simulink library "test"  (Simulink 3.00)
PostLoadFcn:
  | setsysloc simulink_extras
undefined symbols (not defined in the file or in its folder): A, B, C, D, Dd, den, num, offset, sfuncorr, sfunpsd
settings Model: Creator=ldean  LastModifiedBy=jon

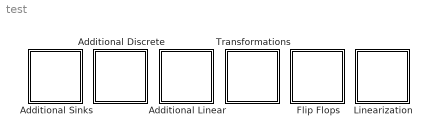
== system test ==
  Additional Discrete : Subsystem
      mask Display: plot([-20 20],[-15 -15],[-15 -15],[-20 20], [ -15  -10  -10 -5 -5  0  0 5 5 10 10 15 15 20],[-10 -10 2  2  13 13 8  8  4  4  1  1  -1 -1])
  Additional Linear : Subsystem
      mask Display: plot([-20 20],[-15 -15],[-15 -15],[-20 20],[-20 20],[-5 18])
  Additional Sinks : Subsystem
      mask Display:
      | plot([-1 1 1 -1 1],[ 1 -1 1 -1 1],[14 4 11 4 6],[14 4 6 4 11],[14 4 11 4 6],[-14 -4 -6 -4 -11],[-14 -4 -11 -4 -6],[14 4 6 4 11],[-14 -4 -11 -4 -6],[-14 -4 -6 -4 -11],
      | [0 0 3 0 -3],[-20 -5 -10 -5 -10],[0 0 3 0 -3],[20 5 10 5 10],[20 5 10 5 10],[0 0 3 0 -3],[-20 -5 -10 -5 -10],[0 0 3 0 -3])
  Flip Flops : Subsystem
  Linearization : Subsystem
  Transformations : Subsystem

== system test/Additional Discrete ==
  Discrete Transfer Fcn (with initial outputs) : Subsystem  mask(Discrete Transfer Function with Initial Outputs){N=[1], D=[1  .5], U0=[1], Y0=-.5, TS=1}
      mask prompts: N "Numerator:"; D "Denominator:"; U0 "Initial input:"; Y0 "Initial output:"; TS "Sample time:"
      mask help: Vector expressions for numerator, and denominator. Coefficients are in descending powers of z.
      mask init:
      | [A,B,C,Dd]=tf2ss(N,D);if (isempty(Y0));[m,n]=size(A);X0=zeros(1,m); end;if (isempty(U0));[m,p]=size(B);U0=zeros(1,p);end;X0=getxo(A,B,C,Dd,U0,Y0,1);
      mask Help: Specify the initial output for the transfer function.  An optimization routine attempts to determine the appropriate initial states so that the specified initial output is achieved.  For more details, see the m-file getxo.m
      mask Display: dpoly(N,D,'z')
  Discrete Transfer Fcn (with initial states) : Subsystem  mask(Discrete Transfer Function with Initial States){N=[1], D=[1  .5], X0=[1], TS=.5}
      mask prompts: N "Numerator:"; D "Denominator:"; X0 "Initial conditions:"; TS "Sample time:"
      mask help: Vector expressions for numerator, and denominator. Coefficients are in descending powers of z.
      mask init:
      | [A,B,C,Dd]=tf2ss(N,D);if (isempty(X0));[m,n]=size(A);X0=zeros(1,m); end;
      mask Help: Specify the initial states for the transfer function.  The state ordering is determined by the m-file tf2ss.  There is no unique mapping of the states in a transfer function to states in a state-space representation.  However, tf2ss will consistently use the same mapping for a given transfer function.
      mask Display: dpoly(N,D,'z')
  Discrete Zero-Pole (with initial outputs) : Subsystem  mask(Discrete Zero-Pole with Initial Outputs){Z=[1], P=[0  .5], K=[1], U0=1, Y0=.5, TS=1}
      mask prompts: Z "Zeros:"; P "Poles:"; K "Gain:"; U0 "Initial input:"; Y0 "Initial output:"; TS "Sample time:"
      mask help: Vector expressions for numerator, denominator, and gain.
      mask init:
      | [A,B,C,D]=zp2ss(Z,P,K);if (isempty(Y0));[m,n]=size(A);X0=zeros(1,m); end;if (isempty(U0));[m,p]=size(B);U0=zeros(1,p);end;X0=getxo(A,B,C,D,U0,Y0,1);
      mask Help: Specify the initial output for the zero-pole-gain system.  An optimization routine attempts to determine the appropriate initial states so that the specified initial output is achieved.  For more details, see the m-file getxo.m
      mask Display: droots(Z,P,K,'z')
  Discrete Zero-Pole (with initial states) : Subsystem  mask(Discrete Zero-Pole with Initial States){Z=[1], P=[0  .5], K=[1], X0=1, TS=.5}
      mask prompts: Z "Zeros:"; P "Poles:"; K "Gain:"; X0 "Initial conditions:"; TS "Sample time:"
      mask help: Vector expressions for numerator, denominator, and gain.
      mask init:
      | [A,B,C,D]=zp2ss(Z,P,K);if (isempty(X0));[m,n]=size(A);X0=zeros(1,m); end;
      mask Help: Specify the initial states for the transfer function.  The state ordering is determined by the m-file zp2ss.  There is no unique mapping of the states in a zero-pole-gain representation to states in a state-space representation.  However, zp2ss will consistently use the same mapping for a given transfer function.
      mask Display: droots(Z,P,K,'z')

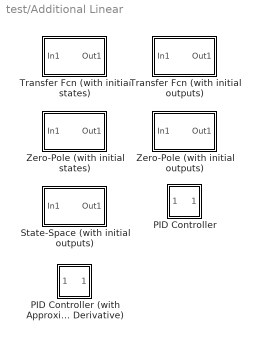
== system test/Additional Linear ==
  PID Controller : Subsystem  mask(PID Controller){P=1, I=1, D=0}
      mask prompts: P "Proportional:"; I "Integral:"; D "Derivative:"
      mask help:
      | Enter expressions for proportional, integral, and derivative terms.
      | P+I/s+Ds
      mask Help: This block implements a PID controller where parameters are entered for the Proportional, Integral and Derivative terms. Unmask this block to see how it works. The derivative term is implemented using a true derivative block.
      mask Display: disp('PID')
  PID Controller (with Approximate Derivative) : Subsystem  mask(PID(2) Controller){P=1, I=1, D=0, N=100}
      mask prompts: P "Proportional:"; I "Integral:"; D "Derivative:"; N "Derivative divisor(N):"
      mask help:
      | Enter Proportional(P), Integral(I), and Derivative(D) and divisor (N) terms.
      | P+I/s+Ds/(1/Ns+1)
      mask Help: This block implements a PID controller where parameters are entered for the Proportional, Integral and Derivative and divisor terms. Unmask this block to see how it works. The derivative term is implemented using an s/(s/N +1)  transfer function block. Making N large can create a "stiff" system.
      mask Display: disp('PID')
  State-Space (with initial outputs) : Subsystem  mask(State-Space with Initial Outputs){A=[-2.0479 -.4517;-.4517 -3.0295], B=[.0591 0]', C=[.2641 .8717], D=0, U0=1, Y0=.5}
      mask prompts: U0 "Initial inputs:"; Y0 "Initial outputs:"
      mask help:
      | State-Space model matrices:
      | dx/dt = Ax + Bu
      | y=Cx +Du
      mask init:
      | if (isempty(Y0));[m,n]=size(A);X0=zeros(1,m); end; if (isempty(U0));[m,p]=size(B);U0=zeros(1,p);end;X0=getxo(A,B,C,D,U0,Y0,0);
      mask Help: Specify an initial output.  An optimization routine is used to attempt to find the steady state x values that satisfy the initial output.  The block states will be initialized to these values.
      mask Display: fprintf('x'' = Ax + Bu\n  y = Cx + Du');
  Transfer Fcn (with initial outputs) : Subsystem  mask(Transfer Function with Initial Outputs){N=[1], D=[1  1], Y0=.5, U0=0}
      mask prompts: N "Numerator:"; D "Denominator:"; Y0 "Initial output:"; U0 "Initial input:"
      mask help: Vector expressions for numerator, and denominator. Coefficients are in descending powers of s.
      mask init:
      | [A,B,C,Dd]=tf2ss(N,D);if (isempty(Y0));[m,n]=size(A);X0=zeros(1,m); end; if (isempty(U0));[m,p]=size(B);U0=zeros(1,p);end;X0=getxo(A,B,C,Dd,U0,Y0,0);
      mask Help: Specify the initial output for the transfer function.  An optimization routine attempts to determine the appropriate initial states so that the specified initial output is achieved.  For more details, see the m-file getxo.m
      mask Display: dpoly(N,D,'s')
  Transfer Fcn (with initial states) : Subsystem  mask(Transfer Function with Initial States){N=[1], D=[1  1], X0=.5}
      mask prompts: N "Numerator:"; D "Denominator:"; X0 "Initial conditions:"
      mask help: Vector expressions for numerator, and denominator. Coefficients are in descending powers of s.
      mask init:
      | [A,B,C,Dd]=tf2ss(N,D);if (isempty(X0));[m,n]=size(A);X0=zeros(1,m); end;
      mask Help: Specify the initial states for the transfer function.  The state ordering is determined by the m-file tf2ss.  There is no unique mapping of the states in a transfer function to states in a state-space representation.  However, tf2ss will consistently use the same mapping for a given transfer function.
      mask Display: dpoly(N,D,'s')
  Zero-Pole (with initial outputs) : Subsystem  mask(Zero-Pole with Initial Outputs){Z=[1], P=[0; -1], K=[1], Y0=.5, U0=0}
      mask prompts: Z "Zeros:"; P "Poles:"; K "Gain:"; Y0 "Initial output:"; U0 "Initial input:"
      mask help: Vector expressions for numerator, denominator, and gain.
      mask init:
      | [A,B,C,D]=zp2ss(Z,P,K);if (isempty(Y0));[m,n]=size(A);X0=zeros(1,m); end; if (isempty(U0));[m,p]=size(B);U0=zeros(1,p);end;X0=getxo(A,B,C,D,U0,Y0,0);
      mask Help: Specify the initial output for the zero-pole-gain system.  An optimization routine attempts to determine the appropriate initial states so that the specified initial output is achieved.  For more details, see the m-file getxo.m
      mask Display: droots(Z,P,K)
  Zero-Pole (with initial states) : Subsystem  mask(Zero-Pole with Initial States){Z=[1], P=[0; -1], K=[1], X0=.5}
      mask prompts: Z "Zeros:"; P "Poles:"; K "Gain:"; X0 "Initial conditions:"
      mask help: Vector expressions for numerator, denominator, and gain.
      mask init:
      | [A,B,C,D]=zp2ss(Z,P,K);if (isempty(X0));[m,n]=size(A);X0=zeros(1,m); end;
      mask Help: Specify the initial states for the transfer function.  The state ordering is determined by the m-file zp2ss.  There is no unique mapping of the states in a zero-pole-gain representation to states in a state-space representation.  However, zp2ss will consistently use the same mapping for a given transfer function.
      mask Display: droots(Z,P,K)

== system test/Additional Sinks ==
  Auto Correlator : Subsystem  LoadFcn=sfuncorr([],[],[],'LoadBlock')  StartFcn=sfuncorr([],[],[],'Start')  mask(Auto Correlator){npts=100, HowOften=50, sampleT=0.1}
      mask prompts: npts "Length of buffer:"; HowOften "Plot after how many points:"; sampleT "Sample time:"
      mask help:
      | Auto correlator using graph window.
      | Requires signal processing toolbox.
      mask init:
      | ts=sampleT(1); if length(sampleT) > 1, offset = sampleT(2);, else, offset = 0; end
      settings: CopyFcn=sfuncorr([],[],[],'CopyBlock')  DeleteFcn=sfuncorr([],[],[],'DeleteBlock')  NameChangeFcn=sfuncorr([],[],[],'NameChange')
      mask Help: This block when hooked to the output of a system displays the auto correlation of the buffer in the graph window. For more see the M-file sfuncorr.
      mask Display: plot(0,0,100,100,[11,93,93,11,11],[90,90,40,40,90],[80,60,40,20],[50,79,50,80])
  Averaging Power Spectral Density : Subsystem  LoadFcn=sfunpsd([],[],[],'LoadBlock')  StartFcn=sfunpsd([],[],[],'Start')  mask(Spectrum Analyzer){npts=128, fftpts=512, HowOften=64, sampleT=0.1}
      mask prompts: npts "Length of buffer:"; fftpts "Number of points for fft:"; HowOften "Plot after how many points:"; sampleT "Sample time:"
      mask help: Spectrum analyzer using graph window.
      mask init:
      | ts=sampleT(1); if length(sampleT) > 1, offset = sampleT(2);, else, offset = 0; end
      settings: CopyFcn=sfunpsd([],[],[],'CopyBlock')  DeleteFcn=sfunpsd([],[],[],'DeleteBlock')  NameChangeFcn=sfunpsd([],[],[],'NameChange')
      mask Help: This block when hooked to the output of a system displays the frequency content of the buffer in the graph window. For more see the M-file sfunpsd.
      mask Display: plot(0,0,100,100,[11,92,92,11,11],[90,90,40,40,90],[82,76,65,57,51,44,35,30,25,20],[65,62,59,63,66,66,67,70,55,50])
  Averaging Spectrum Analyzer : Subsystem  mask(Spectrum Analyzer){npts=256, fftpts=256, HowOften=64, sampleT=0.1}
      mask prompts: npts "Length of buffer:"; fftpts "Number of points for fft:"; HowOften "Plot after how many points:"; sampleT "Sample time:"
      mask help:
      | Spectrum analyser using graph window.
      | Hook input 1 to system input.
      | Hook input 2 to system output.
      mask init:
      | ts=sampleT(1); if length(sampleT) > 1, offset = sampleT(2);, else, offset = 0; end
      mask Help: Hook the system's input to the first port of this block and the system's output to second port. Results are displayed as the frequency response of this system. Use signals with high harmonic content for best results.
      mask Display: plot(0,0,100,100,[12,92,92,12,12],[90,90,40,40,90],[80,72,63,54,47,40,32,20],[61,61,62,65,69,73,75,75])
  Cross Correlator : Subsystem  LoadFcn=sfuncorr([],[],[],'LoadBlock')  StartFcn=sfuncorr([],[],[],'Start')  mask(Cross Correlator){npts=100, HowOften=50, sampleT=0.1}
      mask prompts: npts "Length of buffer:"; HowOften "Plot after how many points:"; sampleT "Sample time:"
      mask help:
      | Cross correlator using graph window.
      | Requires signal processing toolbox.
      mask init:
      | ts=sampleT(1); if length(sampleT) > 1, offset = sampleT(2);, else, offset = 0; end
      settings: CopyFcn=sfuncorr([],[],[],'CopyBlock')  DeleteFcn=sfuncorr([],[],[],'DeleteBlock')  NameChangeFcn=sfuncorr([],[],[],'NameChange')
      mask Help: This block when hooked to the outputs of a system displays the cross correlation of the buffer in the graph window. For more see the M-file sfuncorr.
      mask Display: plot(0,0,100,100,[10,92,92,10,10],[90,90,40,40,90],[80,59,40,20],[70,79,70,79],[79,70,59,51,40,30,21],[60,51,60,50,60,50,60])
  Power Spectral Density : Subsystem  LoadFcn=sfunpsd([],[],[],'LoadBlock')  StartFcn=sfunpsd([],[],[],'Start')  mask(Spectrum Analyzer){npts=128, fftpts=512, HowOften=64, sampleT=0.1}
      mask prompts: npts "Length of buffer:"; fftpts "Number of points for fft:"; HowOften "Plot after how many points:"; sampleT "Sample time:"
      mask help: Spectrum analyser using graph window.
      mask init:
      | ts=sampleT(1); if length(sampleT) > 1, offset = sampleT(2);, else, offset = 0; end
      settings: CopyFcn=sfunpsd([],[],[],'CopyBlock')  DeleteFcn=sfunpsd([],[],[],'DeleteBlock')  NameChangeFcn=sfunpsd([],[],[],'NameChange')
      mask Help: This block when hooked to the output of a system displays the frequency content of the buffer in the graph window. For more see the M-file sfunpsd.
      mask Display: plot(0,0,100,100,[14,91,91,14,14],[86,86,40,40,86],[85,82,80,79,75,67,63,60,57,53,41,36,33,27,24],[49,50,53,50,49,51,54,66,54,50,50,52,81,51,49])
  Spectrum Analyzer : Subsystem  mask(Spectrum Analyzer){npts=256, fftpts=256, HowOften=64, sampleT=0.1}
      mask prompts: npts "Length of buffer:"; fftpts "Number of points for fft:"; HowOften "Plot after how many points:"; sampleT "Sample time:"
      mask help:
      | Spectrum analyser using graph window.
      | Hook input 1 to system input.
      | Hook input 2 to system output.
      mask init:
      | ts=sampleT(1); if length(sampleT) > 1, offset = sampleT(2);, else, offset = 0; end
      mask Help: Hook the system's input to the first port of this block and the system's output to second port. Results are displayed as the frequency response of this system. Use signals with high harmonic content for best results.
      mask Display: plot(0,0,100,100,[11,93,93,11,11],[90,90,40,40,90],[90,80,72,64,55,45,41,36,20],[50,50,52,59,67,75,78,80,80])

== system test/Flip Flops ==
  note: Note: J-K Flip-Flop is Negative-Edge-Triggered
  Clock : Subsystem  mask(Digital clock){@1=2}
      mask prompts: @1 "Period:"
      mask help:
      | Digital clock.
      | Output is set to 1 for the first half of the period.
      mask init:
      | duration = @1/2;
      mask Help: Digital clock for logic systems.
      mask Display: plot(0,0,100,100,[90,75,75,60,60,35,35,20,20,10],[20,20,80,80,19,20,80,80,20,20])
  D Flip-Flop : Subsystem
      mask Type: DFlipFlop
      mask Description: D Flip Flop Block
  D Latch : Subsystem
      mask Type: DLatch
      mask Description: D Latch Flip Flop Block
  J-K Flip-Flop : Subsystem  mask(JKFlipFlop){initial_condition=0}
      mask prompts: initial_condition "Initial condition:"
      mask help: J-K Flip Flop Block (Negative Edge Triggered)
  S-R Flip-Flop : Subsystem  mask(SRFlipFlop){initial_condition=0}
      mask prompts: initial_condition "Initial condition:"
      mask help: S-R Flip Flop Block

== system test/Linearization ==
  note: Block for use with linmod:
  Switched derivative for linearization : Subsystem  mask(Derivative for linearization){switchVal=0, derivConst=100}
      mask prompts: switchVal "Switch value (1 for linearization, 0 for simulation):"; derivConst "Derivative constant  Ns/(s+N):"
      mask help: Switched derivative with proper transfer function approximation for linearization.
      mask init:
      | num = [derivConst,0]; den = [1, derivConst];
      mask Help: This block should be used in place of the derivative when you are linearizing the model. It approximates the derivative with a proper transfer function.
      mask Display: disp('du/dt')
  Switched transport delay for linearization : Subsystem  mask(Delay for linearization.){delay=1, u0=0, switchVal=0, order=2, Npts=1024}
      mask prompts: delay "Time delay:"; u0 "Initial input:"; switchVal "Switch (1 for linearization, 0 for simulation):"; order "Pade order (for linearization):"; Npts "Code generation storage buffer size:"
      mask help:
      | Switched tranpsort delay with pade
      | approximation for linearization.
      mask init:
      | [num, den] = padecoef(delay, order);
      mask Help:
      | This block should be used in place of the transport delay when you are linearizing the model. It uses a pade approximation duirng linearization.
      | See the pade command for more information.
      mask Display: disp('Transport\nDelay')

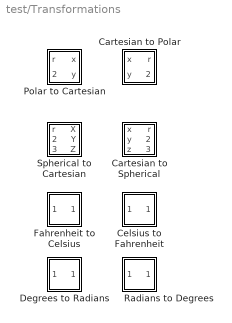
== system test/Transformations ==
  Cartesian to Polar : Subsystem
      mask Type: Cart2Polar
      mask Description:
      | Transformation from cartesian to polar coordinates.
      | [x, y] -> [r, theta]
      | 
      | r = sqrt(x^2 + y^2);
      | theta = atan(y/x);
      mask Help: Unmask this block for more help.
      mask Display: plot(0,0,100,100,[24,20,15,20,20],[85,95,85,95,20],[80,20,95,85,95,85],[70,20,20,15,20,24],[56,56,55,52,50,46],[20,26,31,35,38,42])
  Cartesian to Spherical : Subsystem
      mask Type: Cart2Sph
      mask Description:
      | Transformation from cartesian to spherical coordinates.
      | [x, y, z] -> [r, theta, phi]
      | 
      | p = hypot(x,y); r = hypot(p,z);
      | theta = atan(y/x);
      | phi = atan(p/z);
      mask Help: Unmask this block for more help.
      mask Display: plot(0,0,100,100,[45,40,35,40,40],[85,95,85,95,30],[22,10,14,10,40,95,85,95,85],[12,10,20,10,30,30,25,30,35],[70,40],[80,30],[54,52,50,47,44,40],[53,55,56,58,59,59])
  Celsius to Fahrenheit : Subsystem
      mask Type: CelsiusToFahrenheit
      mask Description:
      | Conversion from degrees Celsius to degrees Fahrenheit.
      | 
      | F=9/5*C+32
      mask Help: This block converts from degrees Celsius to degrees Fahrenheit.
      mask Display: disp('C2F')
  Degrees to Radians : Subsystem
      mask Type: DegreesToRadians
      mask Description:
      | Conversion from Degrees to Radians.
      | 
      | R=pi/180*D
      mask Help: This block converts from Degrees to Radians.
      mask Display: disp('D2R')
  Fahrenheit to Celsius : Subsystem
      mask Type: FahrenheitToCelsius
      mask Description:
      | Conversion from degrees Fahrenheit to degrees Celsius.
      | 
      | C=5/9*(F-32);
      mask Help: This block converts from degrees Fahrenheit to degrees Celsius.
      mask Display: disp('F2C')
  Polar to Cartesian : Subsystem
      mask Type: Polar2Cart
      mask Description:
      | Transformation from polar to cartesian coordinates.
      | [r, theta] -> [x, y]
      | 
      | x = r * cos(theta);
      | y = r * sin(theta);
      mask Help: Unmask this block for more help.
      mask Display: plot(0,0,100,100,[25,20,15,20,20],[85,95,85,95,20],[70,20,95,86,95,85],[60,20,20,15,20,25],[70,70],[45,54],[70,70],[30,40],[70,70],[20,25],[55,65],[60,60],[40,50],[60,60],[25,34],[60,60],[20,21],[60,60],[70,70,68],[57,60,60])
  Radians to Degrees : Subsystem
      mask Type: RadiansToDegrees
      mask Description:
      | Conversion from Radians to Degrees.
      | 
      | D=180/pi*R
      mask Help: This block converts from Radians to Degrees.
      mask Display: disp('R2D')
  Spherical to Cartesian : Subsystem
      mask Type: Sph2Cart
      mask Description:
      | Transformation from spherical to cartesian coordinates.
      | [r, theta, phi] -> [x, y, z]
      | 
      | x = r * sin(phi) * cos(theta);
      | y = r * sin(phi) * sin(theta);
      | z = r * cos(phi);
      mask Help: Unmask this block for more help.
      mask Display: plot(0,0,100,100,[45,40,35,40,40],[85,95,85,95,40],[85,95,85,95,40],[35,40,45,40,40],[60,40,10,20,10,14],[70,40,10,13,10,20],[56,45],[70,70],[60,60],[50,60],[60,60],[30,40],[50,60],[20,20],[30,40],[20,20],[45,55],[35,25],[75,65],[35,25])

== system test/Additional Discrete/Discrete Transfer Fcn (with initial outputs) ==
  In1 : Inport  Port=1  PortWidth=-1  SampleTime=-1  DataType=auto
      settings: SignalType=auto
  Discrete State Space : DiscreteStateSpace  A=A  B=B  C=C  D=Dd  X0=X0  SampleTime=TS
  Out1 : Outport  Port=1  InitialOutput=0
  wires:
  Discrete State Space/1 -> Out1/1
  In1/1 -> Discrete State Space/1

== system test/Additional Discrete/Discrete Transfer Fcn (with initial states) ==
  In1 : Inport  Port=1  PortWidth=-1  SampleTime=-1  DataType=auto
      settings: SignalType=auto
  Discrete State Space : DiscreteStateSpace  A=A  B=B  C=C  D=Dd  X0=X0  SampleTime=TS
  Out1 : Outport  Port=1  InitialOutput=0
  wires:
  Discrete State Space/1 -> Out1/1
  In1/1 -> Discrete State Space/1

== system test/Additional Discrete/Discrete Zero-Pole (with initial outputs) ==
  In1 : Inport  Port=1  PortWidth=-1  SampleTime=-1  DataType=auto
      settings: SignalType=auto
  Discrete State Space : DiscreteStateSpace  A=A  B=B  C=C  D=D  X0=X0  SampleTime=TS
  Out1 : Outport  Port=1  InitialOutput=0
  wires:
  Discrete State Space/1 -> Out1/1
  In1/1 -> Discrete State Space/1

== system test/Additional Discrete/Discrete Zero-Pole (with initial states) ==
  In1 : Inport  Port=1  PortWidth=-1  SampleTime=-1  DataType=auto
      settings: SignalType=auto
  Discrete State Space : DiscreteStateSpace  A=A  B=B  C=C  D=D  X0=X0  SampleTime=TS
  Out1 : Outport  Port=1  InitialOutput=0
  wires:
  Discrete State Space/1 -> Out1/1
  In1/1 -> Discrete State Space/1

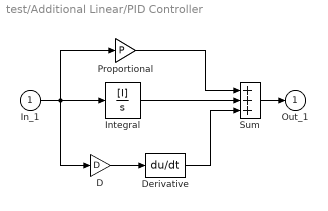
== system test/Additional Linear/PID Controller ==
  In_1 : Inport  Port=1  PortWidth=-1  SampleTime=-1  DataType=auto
      settings: SignalType=auto
  D : Gain  Gain=D  SaturateOnIntegerOverflow=on
  Derivative : Derivative
  Integral : TransferFcn  Numerator=[I]  Denominator=[1 0]
  Proportional : Gain  Gain=P  SaturateOnIntegerOverflow=on
  Sum : Sum  Inputs=+++  SaturateOnIntegerOverflow=on
  Out_1 : Outport  Port=1  InitialOutput=0
  wires:
  D/1 -> Derivative/1
  Sum/1 -> Out_1/1
  In_1/1 -> D/1, Proportional/1, Integral/1
  Derivative/1 -> Sum/3
  Integral/1 -> Sum/2
  Proportional/1 -> Sum/1

== system test/Additional Linear/PID Controller (with Approximate Derivative) ==
  In_1 : Inport  Port=1  PortWidth=-1  SampleTime=-1  DataType=auto
      settings: SignalType=auto
  Derivative : TransferFcn  Numerator=[D, 0]  Denominator=[1/N 1]
  Integral : TransferFcn  Numerator=[I]  Denominator=[1 0]
  Proportional : Gain  Gain=P  SaturateOnIntegerOverflow=on
  Sum : Sum  Inputs=+++  SaturateOnIntegerOverflow=on
  Out_1 : Outport  Port=1  InitialOutput=0
  wires:
  Proportional/1 -> Sum/1
  Integral/1 -> Sum/2
  Derivative/1 -> Sum/3
  In_1/1 -> Proportional/1, Integral/1, Derivative/1
  Sum/1 -> Out_1/1

== system test/Additional Linear/State-Space (with initial outputs) ==
  In1 : Inport  Port=1  PortWidth=-1  SampleTime=-1  DataType=auto
      settings: SignalType=auto
  State-Space : StateSpace  A=A  B=B  C=C  D=D  X0=X0
  Out1 : Outport  Port=1  InitialOutput=0
  wires:
  In1/1 -> State-Space/1
  State-Space/1 -> Out1/1

== system test/Additional Linear/Transfer Fcn (with initial outputs) ==
  In1 : Inport  Port=1  PortWidth=-1  SampleTime=-1  DataType=auto
      settings: SignalType=auto
  State Space : StateSpace  A=A  B=B  C=C  D=Dd  X0=X0
  Out1 : Outport  Port=1  InitialOutput=0
  wires:
  In1/1 -> State Space/1
  State Space/1 -> Out1/1

== system test/Additional Linear/Transfer Fcn (with initial states) ==
  In1 : Inport  Port=1  PortWidth=-1  SampleTime=-1  DataType=auto
      settings: SignalType=auto
  State Space : StateSpace  A=A  B=B  C=C  D=Dd  X0=X0
  Out1 : Outport  Port=1  InitialOutput=0
  wires:
  In1/1 -> State Space/1
  State Space/1 -> Out1/1

== system test/Additional Linear/Zero-Pole (with initial outputs) ==
  In1 : Inport  Port=1  PortWidth=-1  SampleTime=-1  DataType=auto
      settings: SignalType=auto
  State Space : StateSpace  A=A  B=B  C=C  D=D  X0=X0
  Out1 : Outport  Port=1  InitialOutput=0
  wires:
  In1/1 -> State Space/1
  State Space/1 -> Out1/1

== system test/Additional Linear/Zero-Pole (with initial states) ==
  In1 : Inport  Port=1  PortWidth=-1  SampleTime=-1  DataType=auto
      settings: SignalType=auto
  State Space : StateSpace  A=A  B=B  C=C  D=D  X0=X0
  Out1 : Outport  Port=1  InitialOutput=0
  wires:
  In1/1 -> State Space/1
  State Space/1 -> Out1/1

== system test/Additional Sinks/Auto Correlator ==
  input signal : Inport  Port=1  PortWidth=-1  SampleTime=-1  DataType=auto
      settings: SignalType=auto
  sfuncorr : S-Function  FunctionName=sfuncorr  Parameters=npts,HowOften,offset,ts,0,'unbiased'  PortCounts=[]  SFunctionModules=''
  wires:
  input signal/1 -> sfuncorr/1

== system test/Additional Sinks/Averaging Power Spectral Density ==
  input signal : Inport  Port=1  PortWidth=-1  SampleTime=-1  DataType=auto
      settings: SignalType=auto
  sfunpsd : S-Function  FunctionName=sfunpsd  Parameters=fftpts,npts,HowOften,offset,ts,1  PortCounts=[]  SFunctionModules=''
  wires:
  input signal/1 -> sfunpsd/1

== system test/Additional Sinks/Averaging Spectrum Analyzer ==
  system input : Inport  Port=1  PortWidth=-1  SampleTime=-1  DataType=auto
      settings: SignalType=auto
  system output : Inport  Port=2  PortWidth=-1  SampleTime=-1  DataType=auto
      settings: SignalType=auto
  Mux : Mux  Inputs=2
      settings: DisplayOption=none
  sfuntf : S-Function  FunctionName=sfuntf  Parameters=fftpts,npts,HowOften,offset,ts,1  PortCounts=[]  SFunctionModules=''
  wires:
  Mux/1 -> sfuntf/1
  system input/1 -> Mux/1
  system output/1 -> Mux/2

== system test/Additional Sinks/Cross Correlator ==
  signal 1 : Inport  Port=1  PortWidth=-1  SampleTime=-1  DataType=auto
      settings: SignalType=auto
  signal 2 : Inport  Port=2  PortWidth=-1  SampleTime=-1  DataType=auto
      settings: SignalType=auto
  Mux : Mux  Inputs=2
      settings: DisplayOption=none
  sfuncorr : S-Function  FunctionName=sfuncorr  Parameters=npts,HowOften,offset,ts,1,'unbiased'  PortCounts=[]  SFunctionModules=''
  wires:
  signal 1/1 -> Mux/1
  signal 2/1 -> Mux/2
  Mux/1 -> sfuncorr/1

== system test/Additional Sinks/Power Spectral Density ==
  input signal : Inport  Port=1  PortWidth=-1  SampleTime=-1  DataType=auto
      settings: SignalType=auto
  sfunpsd : S-Function  FunctionName=sfunpsd  Parameters=fftpts,npts,HowOften,offset,ts,0  PortCounts=[]  SFunctionModules=''
  wires:
  input signal/1 -> sfunpsd/1

== system test/Additional Sinks/Spectrum Analyzer ==
  system input : Inport  Port=1  PortWidth=-1  SampleTime=-1  DataType=auto
      settings: SignalType=auto
  system output : Inport  Port=2  PortWidth=-1  SampleTime=-1  DataType=auto
      settings: SignalType=auto
  Mux : Mux  Inputs=2
      settings: DisplayOption=none
  sfuntf : S-Function  FunctionName=sfuntf  Parameters=fftpts,npts,HowOften,offset,ts,0  PortCounts=[]  SFunctionModules=''
  wires:
  system output/1 -> Mux/2
  system input/1 -> Mux/1
  Mux/1 -> sfuntf/1

== system test/Flip Flops/Clock ==
  Constant : Constant  Value=1
  Sum : Sum  Inputs=+-  SaturateOnIntegerOverflow=on
  Unit Delay : UnitDelay  Orientation=left  X0=0  SampleTime=duration
  out_1 : Outport  Port=1  InitialOutput=0
  wires:
  Unit Delay/1 -> Sum/2
  Sum/1 -> out_1/1, Unit Delay/1
  Constant/1 -> Sum/1

== system test/Flip Flops/D Flip-Flop ==
  D : Inport  Port=1  PortWidth=-1  SampleTime=-1  DataType=auto
      settings: SignalType=auto
  CLK : Inport  Orientation=down  Port=2  PortWidth=-1  SampleTime=-1  DataType=auto
      settings: SignalType=auto
  !CLR : Inport  Orientation=down  Port=3  PortWidth=-1  SampleTime=-1  DataType=auto
      settings: SignalType=auto
  D Flip-Flop : Subsystem
  Q : Outport  Port=1  InitialOutput=0
  !Q : Outport  Port=2  InitialOutput=1
  wires:
  CLK/1 -> D Flip-Flop/Trigger
  !CLR/1 -> D Flip-Flop/Enable
  D Flip-Flop/1(Q) -> Q/1
  D/1 -> D Flip-Flop/1(D)
  D Flip-Flop/2(!Q) -> !Q/1

== system test/Flip Flops/D Latch ==
  D : Inport  Port=1  PortWidth=-1  SampleTime=-1  DataType=auto
      settings: SignalType=auto
  C : Inport  Orientation=down  Port=2  PortWidth=-1  SampleTime=-1  DataType=auto
      settings: SignalType=auto
  D Latch : Subsystem
  Q : Outport  Port=1  InitialOutput=0
  !Q : Outport  Port=2  InitialOutput=1
  wires:
  D Latch/2(!Q) -> !Q/1
  D/1 -> D Latch/1(D)
  D Latch/1(Q) -> Q/1
  C/1 -> D Latch/Enable

== system test/Flip Flops/J-K Flip-Flop ==
  J : Inport  Port=1  PortWidth=-1  SampleTime=-1  DataType=auto
      settings: SignalType=auto
  CLK : Inport  Orientation=down  Port=2  PortWidth=-1  SampleTime=-1  DataType=auto
      settings: SignalType=auto
  K : Inport  Port=3  PortWidth=-1  SampleTime=-1  DataType=auto
      settings: SignalType=auto
  J-K Flip-Flop : Subsystem
  Q : Outport  Port=1
  !Q : Outport  Port=2
  wires:
  J-K Flip-Flop/2(!Q) -> !Q/1
  K/1 -> J-K Flip-Flop/2(K)
  J/1 -> J-K Flip-Flop/1(J)
  J-K Flip-Flop/1(Q) -> Q/1
  CLK/1 -> J-K Flip-Flop/Trigger

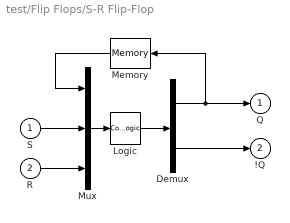
== system test/Flip Flops/S-R Flip-Flop ==
  S : Inport  Port=1  PortWidth=-1  SampleTime=-1  DataType=auto
      settings: SignalType=auto
  R : Inport  Port=2  PortWidth=-1  SampleTime=-1  DataType=auto
      settings: SignalType=auto
  Demux : Demux  Outputs=2
  Logic : CombinatorialLogic  TruthTable=[0 1;0 1;1 0;0 1;1 0;0 1;1 0;1 0]
  Memory : Memory  Orientation=left  X0=initial_condition  InheritSampleTime=on
  Mux : Mux  Inputs=3
      settings: DisplayOption=none
  Q : Outport  Port=1  InitialOutput=0
  !Q : Outport  Port=2  InitialOutput=1
  wires:
  R/1 -> Mux/3
  S/1 -> Mux/2
  Memory/1 -> Mux/1
  Demux/1 -> Memory/1, Q/1
  Demux/2 -> !Q/1
  Logic/1 -> Demux/1
  Mux/1 -> Logic/1

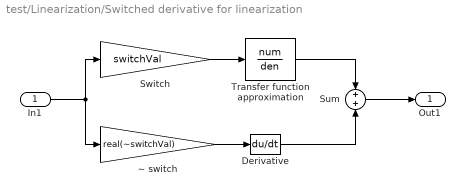
== system test/Linearization/Switched derivative for linearization ==
  In1 : Inport  Port=1  PortWidth=-1  SampleTime=-1  DataType=auto
      settings: SignalType=auto
  Derivative : Derivative
  Sum : Sum  Inputs=++  SaturateOnIntegerOverflow=on
  Switch : Gain  Gain=switchVal  SaturateOnIntegerOverflow=on
  Transfer function approximation : TransferFcn  Numerator=num  Denominator=den
  ~ switch : Gain  Gain=real(~switchVal)  SaturateOnIntegerOverflow=on
  Out1 : Outport  Port=1
  wires:
  In1/1 -> ~ switch/1, Switch/1
  Switch/1 -> Transfer function approximation/1
  ~ switch/1 -> Derivative/1
  Derivative/1 -> Sum/2
  Transfer function approximation/1 -> Sum/1
  Sum/1 -> Out1/1

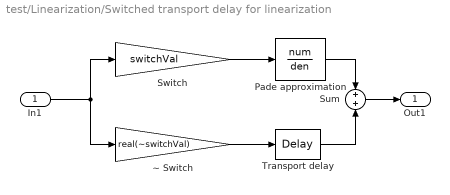
== system test/Linearization/Switched transport delay for linearization ==
  In1 : Inport  Port=1  PortWidth=-1  SampleTime=-1  DataType=auto
      settings: SignalType=auto
  Pade approximation : TransferFcn  Numerator=num  Denominator=den
  Sum : Sum  Inputs=++  SaturateOnIntegerOverflow=on
  Switch : Gain  Gain=switchVal  SaturateOnIntegerOverflow=on
  Transport delay : TransportDelay  DelayTime=delay  InitialInput=u0  BufferSize=Npts
  ~ Switch : Gain  Gain=real(~switchVal)  SaturateOnIntegerOverflow=on
  Out1 : Outport  Port=1
  wires:
  ~ Switch/1 -> Transport delay/1
  Switch/1 -> Pade approximation/1
  Transport delay/1 -> Sum/2
  Pade approximation/1 -> Sum/1
  Sum/1 -> Out1/1
  In1/1 -> ~ Switch/1, Switch/1

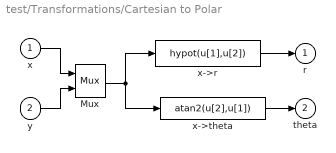
== system test/Transformations/Cartesian to Polar ==
  x : Inport  Port=1  PortWidth=-1  SampleTime=-1  DataType=auto
      settings: SignalType=auto
  y : Inport  Port=2  PortWidth=-1  SampleTime=-1  DataType=auto
      settings: SignalType=auto
  Mux : Mux  Inputs=2
      settings: DisplayOption=none
  x->r : Fcn  Expr=hypot(u[1],u[2])
  x->theta : Fcn  Expr=atan2(u[2],u[1])
  r : Outport  Port=1  InitialOutput=0
  theta : Outport  Port=2  InitialOutput=0
  wires:
  x->theta/1 -> theta/1
  y/1 -> Mux/2
  x/1 -> Mux/1
  x->r/1 -> r/1
  Mux/1 -> x->r/1, x->theta/1

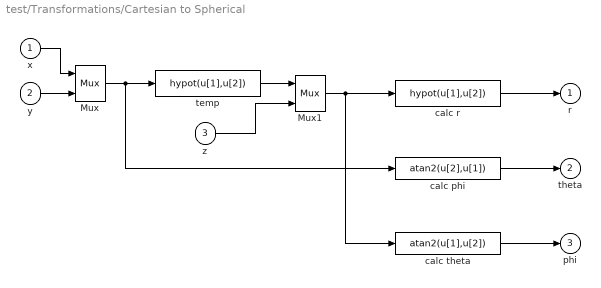
== system test/Transformations/Cartesian to Spherical ==
  x : Inport  Port=1  PortWidth=-1  SampleTime=-1  DataType=auto
      settings: SignalType=auto
  y : Inport  Port=2  PortWidth=-1  SampleTime=-1  DataType=auto
      settings: SignalType=auto
  z : Inport  Port=3  PortWidth=-1  SampleTime=-1  DataType=auto
      settings: SignalType=auto
  Mux : Mux  Inputs=2
      settings: DisplayOption=none
  Mux1 : Mux  Inputs=2
      settings: DisplayOption=none
  calc phi : Fcn  Expr=atan2(u[2],u[1])
  calc r : Fcn  Expr=hypot(u[1],u[2])
  calc theta : Fcn  Expr=atan2(u[1],u[2])
  temp : Fcn  Expr=hypot(u[1],u[2])
  "r " : Outport  Port=1  InitialOutput=0
  theta : Outport  Port=2  InitialOutput=0
  phi : Outport  Port=3  InitialOutput=0
  wires:
  Mux1/1 -> calc r/1, calc theta/1
  Mux/1 -> temp/1, calc phi/1
  calc r/1 -> "r "/1
  z/1 -> Mux1/2
  temp/1 -> Mux1/1
  x/1 -> Mux/1
  y/1 -> Mux/2
  calc theta/1 -> phi/1
  calc phi/1 -> theta/1

== system test/Transformations/Celsius to Fahrenheit ==
  Celsius in : Inport  Port=1  PortWidth=-1  SampleTime=-1  DataType=auto
      settings: SignalType=auto
  Constant : Constant  Value=32
  Gain : Gain  Gain=9/5  SaturateOnIntegerOverflow=on
  Sum : Sum  Inputs=++  SaturateOnIntegerOverflow=on
  Fahrenheit out : Outport  Port=1  InitialOutput=0
  wires:
  Constant/1 -> Sum/2
  Sum/1 -> Fahrenheit out/1
  Gain/1 -> Sum/1
  Celsius in/1 -> Gain/1

== system test/Transformations/Degrees to Radians ==
  Degrees in : Inport  Port=1  PortWidth=-1  SampleTime=-1  DataType=auto
      settings: SignalType=auto
  Gain1 : Gain  Gain=pi/180  SaturateOnIntegerOverflow=on
  Radians out : Outport  Port=1  InitialOutput=0
  wires:
  Degrees in/1 -> Gain1/1
  Gain1/1 -> Radians out/1

== system test/Transformations/Fahrenheit to Celsius ==
  Fahrenheit in : Inport  Port=1  PortWidth=-1  SampleTime=-1  DataType=auto
      settings: SignalType=auto
  Constant : Constant  Value=32
  Gain1 : Gain  Gain=5/9  SaturateOnIntegerOverflow=on
  Sum : Sum  Inputs=+-  SaturateOnIntegerOverflow=on
  Celsius out : Outport  Port=1  InitialOutput=0
  wires:
  Gain1/1 -> Celsius out/1
  Sum/1 -> Gain1/1
  Fahrenheit in/1 -> Sum/1
  Constant/1 -> Sum/2

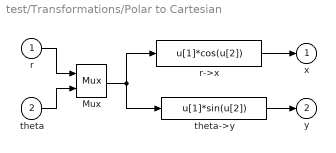
== system test/Transformations/Polar to Cartesian ==
  "r " : Inport  Port=1  PortWidth=-1  SampleTime=-1  DataType=auto
      settings: SignalType=auto
  "theta " : Inport  Port=2  PortWidth=-1  SampleTime=-1  DataType=auto
      settings: SignalType=auto
  Mux : Mux  Inputs=2
      settings: DisplayOption=none
  r->x : Fcn  Expr=u[1]*cos(u[2])
  theta->y : Fcn  Expr=u[1]*sin(u[2])
  x : Outport  Port=1  InitialOutput=0
  y : Outport  Port=2  InitialOutput=0
  wires:
  Mux/1 -> r->x/1, theta->y/1
  r->x/1 -> x/1
  "r "/1 -> Mux/1
  "theta "/1 -> Mux/2
  theta->y/1 -> y/1

== system test/Transformations/Radians to Degrees ==
  Radians in : Inport  Port=1  PortWidth=-1  SampleTime=-1  DataType=auto
      settings: SignalType=auto
  Gain : Gain  Gain=180/pi  SaturateOnIntegerOverflow=on
  Degrees out : Outport  Port=1  InitialOutput=0
  wires:
  Radians in/1 -> Gain/1
  Gain/1 -> Degrees out/1

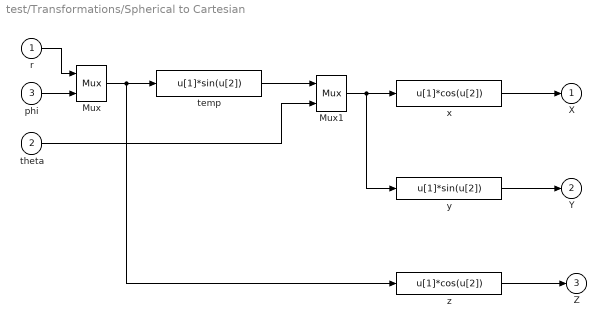
== system test/Transformations/Spherical to Cartesian ==
  r : Inport  Port=1  PortWidth=-1  SampleTime=-1  DataType=auto
      settings: SignalType=auto
  theta : Inport  Port=2  PortWidth=-1  SampleTime=-1  DataType=auto
      settings: SignalType=auto
  phi : Inport  Port=3  PortWidth=-1  SampleTime=-1  DataType=auto
      settings: SignalType=auto
  Mux : Mux  Inputs=2
      settings: DisplayOption=none
  Mux1 : Mux  Inputs=2
      settings: DisplayOption=none
  temp : Fcn  Expr=u[1]*sin(u[2])
  x : Fcn  Expr=u[1]*cos(u[2])
  y : Fcn  Expr=u[1]*sin(u[2])
  z : Fcn  Expr=u[1]*cos(u[2])
  X : Outport  Port=1  InitialOutput=0
  Y : Outport  Port=2  InitialOutput=0
  Z : Outport  Port=3  InitialOutput=0
  wires:
  Mux/1 -> temp/1, z/1
  Mux1/1 -> x/1, y/1
  theta/1 -> Mux1/2
  phi/1 -> Mux/2
  r/1 -> Mux/1
  temp/1 -> Mux1/1
  x/1 -> X/1
  y/1 -> Y/1
  z/1 -> Z/1

== system test/Flip Flops/D Flip-Flop/D Flip-Flop ==
  D : Inport  Port=1  PortWidth=-1  SampleTime=-1  DataType=auto
      settings: SignalType=auto
  C : EnablePort
  Trigger : TriggerPort  TriggerType=rising  OutputDataType=auto
  Logic : Logic  Operator=NOT  Inputs=1
  Q : Outport  Port=1  OutputWhenDisabled=reset  InitialOutput=0
  !Q : Outport  Port=2  OutputWhenDisabled=reset  InitialOutput=1
  wires:
  Logic/1 -> !Q/1
  D/1 -> Q/1, Logic/1

== system test/Flip Flops/D Latch/D Latch ==
  D : Inport  Port=1  PortWidth=-1  SampleTime=-1  DataType=auto
      settings: SignalType=auto
  C : EnablePort
  Logic : Logic  Operator=NOT  Inputs=1
  Q : Outport  Port=1  InitialOutput=0
  !Q : Outport  Port=2  InitialOutput=1
  wires:
  D/1 -> Logic/1, Q/1
  Logic/1 -> !Q/1

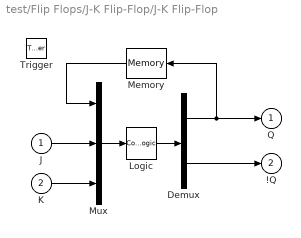
== system test/Flip Flops/J-K Flip-Flop/J-K Flip-Flop ==
  J : Inport  Port=1  PortWidth=-1  SampleTime=-1  DataType=auto
      settings: SignalType=auto
  K : Inport  Port=2  PortWidth=-1  SampleTime=-1  DataType=auto
      settings: SignalType=auto
  Trigger : TriggerPort  TriggerType=falling  OutputDataType=auto
  Demux : Demux  Outputs=2
  Logic : CombinatorialLogic  TruthTable=[0 1; 0 1; 1 0; 1 0; 1 0; 0 1; 1 0; 0 1]
  Memory : Memory  Orientation=left  X0=initial_condition  InheritSampleTime=on
  Mux : Mux  Inputs=3
  Q : Outport  Port=1  InitialOutput=initial_condition
  !Q : Outport  Port=2  InitialOutput=~initial_condition
  wires:
  J/1 -> Mux/2
  K/1 -> Mux/3
  Memory/1 -> Mux/1
  Demux/1 -> Q/1, Memory/1
  Demux/2 -> !Q/1
  Logic/1 -> Demux/1
  Mux/1 -> Logic/1
